simulink library "autolibshared"  (R2019b)
settings: Solver=ode45  StartTime=0.0  StopTime=10.0  RelTol=1e-3  EnableMultiTasking=on
undefined symbols (not defined in the file or in its folder): AccelCycle, aMode, DriveCycle, GearCycle, psi, x_o
libraries: autolibsharedcommon x20, $bdroot x7, autolibutils x2, autolibpowerinfoutils x1
(part 3 of 4)

== system autolibshared/Longitudinal Wheel/Longitudinal Parameters/Magic Formula Peak Value ==
  TirePrs : Inport
  Longitudinal Scaling : Inport  Port=2
  Bus Creator : BusCreator  Inputs=3
  Bus Creator1 : BusCreator  Inputs=5
  Bus Creator2 : BusCreator  Inputs=1
  Constant : Constant  Value=D
  Constant1 : Constant  Value=C
  Constant12 : Constant  Value=zeros(1,3)
  Constant14 : Constant  Value=zeros(3,3)
  Constant19 : Constant  Value=zeros(1,3)
  Constant2 : Constant  Value=zeros(34,1)
  Constant6 : Constant  Value=E
  Constant7 : Constant  Value=B
  Terminator : Terminator
  Magic Peak : Outport  VectorParamsAs1DForOutWhenUnconnected=off
  Magic Load Varying Fxo : Outport  Port=2  VectorParamsAs1DForOutWhenUnconnected=off
  Mapped Longitudinal Force : Outport  Port=3  VectorParamsAs1DForOutWhenUnconnected=off
  wires:
  Constant2/1 -> Bus Creator2/1
  Bus Creator2/1 -> Magic Load Varying Fxo/1
  Constant19/1 -> Bus Creator/1  "kappaFx"
  Constant12/1 -> Bus Creator/2  "FzFx"
  Constant14/1 -> Bus Creator/3  "FxMap"
  Longitudinal Scaling/1 -> Bus Creator1/5  "lam_mux"
  Bus Creator1/1 -> Magic Peak/1
  Bus Creator/1 -> Mapped Longitudinal Force/1  "mappedFx"
  Constant/1 -> Bus Creator1/1  "D"
  Constant1/1 -> Bus Creator1/2  "C"
  Constant6/1 -> Bus Creator1/4  "E"
  Constant7/1 -> Bus Creator1/3  "B"
  TirePrs/1 -> Terminator/1  "TirePrs"

== system autolibshared/Longitudinal Wheel/Longitudinal Parameters/Mapped Force ==
  TirePrs : Inport
  Longitudinal Scaling : Inport  Port=2
  Bus Creator : BusCreator  Inputs=3
  Bus Creator1 : BusCreator  Inputs=5
  Bus Creator2 : BusCreator  Inputs=1
  Constant{,1,6..7} (4 alike) : Constant  Value=0
  Constant12 : Constant  Value=FzFx
  Constant14 : Constant  Value=FxMap
  Constant19 : Constant  Value=kappaFx
  Constant2 : Constant  Value=zeros(34,1)
  Terminator : Terminator
  Magic Peak : Outport  VectorParamsAs1DForOutWhenUnconnected=off
  Magic Load Varying Fxo : Outport  Port=2  VectorParamsAs1DForOutWhenUnconnected=off
  Mapped Longitudinal Force : Outport  Port=3  VectorParamsAs1DForOutWhenUnconnected=off
  wires:
  Bus Creator2/1 -> Magic Load Varying Fxo/1
  Constant2/1 -> Bus Creator2/1
  Longitudinal Scaling/1 -> Bus Creator1/5  "lam_mux"
  Constant/1 -> Bus Creator1/1  "D"
  Constant6/1 -> Bus Creator1/4  "E"
  Bus Creator1/1 -> Magic Peak/1
  Constant7/1 -> Bus Creator1/3  "B"
  Constant1/1 -> Bus Creator1/2  "C"
  Constant19/1 -> Bus Creator/1  "kappaFx"
  Constant12/1 -> Bus Creator/2  "FzFx"
  Constant14/1 -> Bus Creator/3  "FxMap"
  Bus Creator/1 -> Mapped Longitudinal Force/1  "mappedFx"
  TirePrs/1 -> Terminator/1  "TirePrs"

== system autolibshared/Longitudinal Wheel/Rolling Parameters/ISO ==
  note: 8
  note: 16
  Temp : Inport  Unit=K
  Bus Creator : BusCreator  Inputs=3
  Bus Creator1 : BusCreator  Inputs=16
  Constant1 : Constant  Value=TMIN
  Constant{2,5,7,9..11,17..18} (8 alike) : Constant  Value=0
  Constant12 : Constant  Value=zeros(1,3)
  Constant13 : Constant  Value=Fpl
  Constant14 : Constant  Value=zeros(3,3)
  Constant15 : Constant  Value=Kt
  Constant16 : Constant  Value=Tmeas
  Constant19 : Constant  Value=zeros(1,3)
  Constant3 : Constant  Value=TMAX
  Constant4 : Constant  Value=UNLOADED_RADIUS
  Constant8 : Constant  Value=Cr
  Signal Specification{,1..3} (4 alike) : SignalSpecification  Unit=degC
  Signal Specification4 : SignalSpecification  Unit=K
  Signal Specification5 : SignalSpecification  Unit=K
  Signal Specification6 : SignalSpecification  Unit=K
  Unit Conversion{,1..3} (4 alike) : UnitConversion
  Magic Rolling Resistance : Outport  VectorParamsAs1DForOutWhenUnconnected=off
  Mapped Rolling Resistance : Outport  Port=2  VectorParamsAs1DForOutWhenUnconnected=off
  wires:
  Unit Conversion/1 -> Signal Specification/1
  Temp/1 -> Unit Conversion/1  "Temp"
  Constant10/1 -> Bus Creator1/13  "lam_My"
  Bus Creator1/1 -> Magic Rolling Resistance/1
  Constant18/1 -> Bus Creator1/11  "QSY8"
  Constant15/1 -> Bus Creator1/6  "QSY3"
  Constant17/1 -> Bus Creator1/10  "QSY7"
  Constant8/1 -> Bus Creator1/5  "QSY2"
  Constant5/1 -> Bus Creator1/2  "FNOMIN"
  Constant13/1 -> Bus Creator1/4  "QSY1"
  Constant2/1 -> Bus Creator1/3  "NOMPRES"
  Constant4/1 -> Bus Creator1/14  "UNLOADED_RADIUS"
  Signal Specification/1 -> Bus Creator1/1  "TAmb"
  Constant7/1 -> Bus Creator1/8  "QSY5"
  Constant9/1 -> Bus Creator1/9  "QSY6"
  Constant11/1 -> Bus Creator1/12  "gamma"
  Bus Creator/1 -> Mapped Rolling Resistance/1  "mappedMy"
  Constant14/1 -> Bus Creator/3  "MyMap"
  Constant12/1 -> Bus Creator/2  "FzMy"
  Constant19/1 -> Bus Creator/1  "VxMy"
  Unit Conversion1/1 -> Signal Specification1/1
  Signal Specification1/1 -> Bus Creator1/15  "TMin"
  Constant1/1 -> Signal Specification5/1
  Unit Conversion2/1 -> Signal Specification2/1
  Signal Specification2/1 -> Bus Creator1/16  "Tmax"
  Constant3/1 -> Signal Specification6/1
  Unit Conversion3/1 -> Signal Specification3/1
  Constant16/1 -> Signal Specification4/1
  Signal Specification3/1 -> Bus Creator1/7  "Tmeas"
  Signal Specification4/1 -> Unit Conversion3/1
  Signal Specification5/1 -> Unit Conversion1/1
  Signal Specification6/1 -> Unit Conversion2/1

== system autolibshared/Longitudinal Wheel/Rolling Parameters/Magic ==
  note: 8
  note: 16
  TirePrs : Inport  Unit=Pa
  Bus Creator : BusCreator  Inputs=3
  Bus Creator1 : BusCreator  Inputs=16
  Constant1 : Constant  Value=PRESMIN
  Constant10 : Constant  Value=lam_My
  Constant11 : Constant  Value=gamma
  Constant12 : Constant  Value=zeros(1,3)
  Constant13 : Constant  Value=QSY1
  Constant14 : Constant  Value=zeros(3,3)
  Constant15 : Constant  Value=QSY3
  Constant16 : Constant  Value=QSY4
  Constant17 : Constant  Value=QSY7
  Constant18 : Constant  Value=QSY8
  Constant19 : Constant  Value=zeros(1,3)
  Constant2 : Constant  Value=NOMPRES
  Constant3 : Constant  Value=PRESMAX
  Constant4 : Constant  Value=UNLOADED_RADIUS
  Constant5 : Constant  Value=FNOMIN
  Constant7 : Constant  Value=QSY5
  Constant8 : Constant  Value=QSY2
  Constant9 : Constant  Value=QSY6
  Magic Rolling Resistance : Outport  VectorParamsAs1DForOutWhenUnconnected=off
  Mapped Rolling Resistance : Outport  Port=2  VectorParamsAs1DForOutWhenUnconnected=off
  wires:
  Constant19/1 -> Bus Creator/1  "VxMy"
  Constant12/1 -> Bus Creator/2  "FzMy"
  Constant14/1 -> Bus Creator/3  "MyMap"
  Bus Creator/1 -> Mapped Rolling Resistance/1  "mappedMy"
  Constant11/1 -> Bus Creator1/12  "gamma"
  Constant9/1 -> Bus Creator1/9  "QSY6"
  Constant7/1 -> Bus Creator1/8  "QSY5"
  TirePrs/1 -> Bus Creator1/1  "TirePrs"
  Constant4/1 -> Bus Creator1/14  "UNLOADED_RADIUS"
  Constant3/1 -> Bus Creator1/16  "PRESMAX"
  Constant1/1 -> Bus Creator1/15  "PRESMIN"
  Constant2/1 -> Bus Creator1/3  "NOMPRES"
  Constant13/1 -> Bus Creator1/4  "QSY1"
  Constant5/1 -> Bus Creator1/2  "FNOMIN"
  Constant8/1 -> Bus Creator1/5  "QSY2"
  Constant17/1 -> Bus Creator1/10  "QSY7"
  Constant15/1 -> Bus Creator1/6  "QSY3"
  Constant16/1 -> Bus Creator1/7  "QSY4"
  Constant18/1 -> Bus Creator1/11  "QSY8"
  Bus Creator1/1 -> Magic Rolling Resistance/1
  Constant10/1 -> Bus Creator1/13  "lam_My"

== system autolibshared/Longitudinal Wheel/Rolling Parameters/Mapped ==
  TirePrs : Inport  Unit=Pa
  Bus Creator : BusCreator  Inputs=3
  Bus Creator1 : BusCreator  Inputs=16
  Constant{1..10,13,15..18} (15 alike) : Constant  Value=0
  Constant12 : Constant  Value=FzMy
  Constant14 : Constant  Value=MyMap
  Constant19 : Constant  Value=VxMy
  Magic Rolling Resistance : Outport  VectorParamsAs1DForOutWhenUnconnected=off
  Mapped Rolling Resistance : Outport  Port=2  VectorParamsAs1DForOutWhenUnconnected=off
  wires:
  Constant19/1 -> Bus Creator/1  "VxMy"
  Constant12/1 -> Bus Creator/2  "FzMy"
  Constant14/1 -> Bus Creator/3  "MyMap"
  Bus Creator/1 -> Mapped Rolling Resistance/1  "mappedMy"
  Constant6/1 -> Bus Creator1/12  "gamma"
  Constant9/1 -> Bus Creator1/9  "QSY6"
  Constant7/1 -> Bus Creator1/8  "QSY5"
  TirePrs/1 -> Bus Creator1/1  "TirePrs"
  Constant4/1 -> Bus Creator1/14  "UNLOADED_RADIUS"
  Constant3/1 -> Bus Creator1/16  "PRESMAX"
  Constant1/1 -> Bus Creator1/15  "PRESMIN"
  Constant2/1 -> Bus Creator1/3  "NOMPRES"
  Constant13/1 -> Bus Creator1/4  "QSY1"
  Constant5/1 -> Bus Creator1/2  "FNOMIN"
  Constant8/1 -> Bus Creator1/5  "QSY2"
  Constant17/1 -> Bus Creator1/10  "QSY7"
  Constant15/1 -> Bus Creator1/6  "QSY3"
  Constant16/1 -> Bus Creator1/7  "QSY4"
  Constant18/1 -> Bus Creator1/11  "QSY8"
  Bus Creator1/1 -> Magic Rolling Resistance/1
  Constant10/1 -> Bus Creator1/13  "lam_My"

== system autolibshared/Longitudinal Wheel/Rolling Parameters/None ==
  Bus Creator : BusCreator  Inputs=3
  Bus Creator1 : BusCreator  Inputs=16
  Constant{1,4,6..9,11,13,15..16} (10 alike) : Constant  Value=0
  Constant{2..3,5,10,17..18} (6 alike) : Constant
  Constant12 : Constant  Value=zeros(1,3)
  Constant14 : Constant  Value=zeros(3,3)
  Constant19 : Constant  Value=zeros(1,3)
  Magic Rolling Resistance : Outport  VectorParamsAs1DForOutWhenUnconnected=off
  Mapped Rolling Resistance : Outport  Port=2  VectorParamsAs1DForOutWhenUnconnected=off
  wires:
  Constant19/1 -> Bus Creator/1  "VxMy"
  Constant12/1 -> Bus Creator/2  "FzMy"
  Constant14/1 -> Bus Creator/3  "MyMap"
  Bus Creator/1 -> Mapped Rolling Resistance/1  "mappedMy"
  Constant6/1 -> Bus Creator1/12  "gamma"
  Constant9/1 -> Bus Creator1/9  "QSY6"
  Constant7/1 -> Bus Creator1/8  "QSY5"
  Constant11/1 -> Bus Creator1/1  "TirePrs"
  Constant4/1 -> Bus Creator1/14  "UNLOADED_RADIUS"
  Constant3/1 -> Bus Creator1/16  "PRESMAX"
  Constant1/1 -> Bus Creator1/15  "PRESMIN"
  Constant2/1 -> Bus Creator1/3  "NOMPRES"
  Constant13/1 -> Bus Creator1/4  "QSY1"
  Constant5/1 -> Bus Creator1/2  "FNOMIN"
  Constant8/1 -> Bus Creator1/5  "QSY2"
  Constant17/1 -> Bus Creator1/10  "QSY7"
  Constant15/1 -> Bus Creator1/6  "QSY3"
  Constant16/1 -> Bus Creator1/7  "QSY4"
  Constant18/1 -> Bus Creator1/11  "QSY8"
  Bus Creator1/1 -> Magic Rolling Resistance/1
  Constant10/1 -> Bus Creator1/13  "lam_My"

== system autolibshared/Longitudinal Wheel/Rolling Parameters/Simple ==
  note: 16
  note: 8
  TirePrs : Inport  Unit=Pa
  Bus Creator : BusCreator  Inputs=3
  Bus Creator1 : BusCreator  Inputs=16
  Constant1 : Constant  Value=PRESMIN
  Constant{2,5,7,9..11,16} (7 alike) : Constant  Value=0
  Constant12 : Constant  Value=zeros(1,3)
  Constant13 : Constant  Value=aMy
  Constant14 : Constant  Value=zeros(3,3)
  Constant15 : Constant  Value=cMy
  Constant17 : Constant  Value=betaMy
  Constant18 : Constant  Value=alphaMy
  Constant19 : Constant  Value=zeros(1,3)
  Constant3 : Constant  Value=PRESMAX
  Constant4 : Constant  Value=UNLOADED_RADIUS
  Constant8 : Constant  Value=bMy
  Magic Rolling Resistance : Outport  VectorParamsAs1DForOutWhenUnconnected=off
  Mapped Rolling Resistance : Outport  Port=2  VectorParamsAs1DForOutWhenUnconnected=off
  wires:
  Constant19/1 -> Bus Creator/1  "VxMy"
  Constant12/1 -> Bus Creator/2  "FzMy"
  Constant14/1 -> Bus Creator/3  "MyMap"
  Bus Creator/1 -> Mapped Rolling Resistance/1  "mappedMy"
  Constant11/1 -> Bus Creator1/12  "gamma"
  Constant9/1 -> Bus Creator1/9  "QSY6"
  Constant7/1 -> Bus Creator1/8  "QSY5"
  TirePrs/1 -> Bus Creator1/1  "TirePrs"
  Constant4/1 -> Bus Creator1/14  "UNLOADED_RADIUS"
  Constant3/1 -> Bus Creator1/16  "PRESMAX"
  Constant1/1 -> Bus Creator1/15  "PRESMIN"
  Constant2/1 -> Bus Creator1/3  "NOMPRES"
  Constant13/1 -> Bus Creator1/4  "QSY1"
  Constant5/1 -> Bus Creator1/2  "FNOMIN"
  Constant8/1 -> Bus Creator1/5  "QSY2"
  Constant17/1 -> Bus Creator1/10  "QSY7"
  Constant15/1 -> Bus Creator1/6  "QSY3"
  Constant16/1 -> Bus Creator1/7  "QSY4"
  Constant18/1 -> Bus Creator1/11  "QSY8"
  Bus Creator1/1 -> Magic Rolling Resistance/1
  Constant10/1 -> Bus Creator1/13  "lam_My"

== system autolibshared/Longitudinal Wheel/Vertical DOF/Magic Vertical DOF ==
  Fz : Inport
  Ground : Inport  Port=2
  FzTire : Inport  Port=3
  TirePrs : Inport  Port=4
  Bus Creator1 : BusCreator  Inputs=24
  Constant1 : Constant  Value=PRESMIN
  Constant10 : Constant  Value=Q_FCY
  Constant11 : Constant  Value=Q_FCY2
  Constant13 : Constant  Value=Q_CAM
  Constant14 : Constant  Value=NOMPRES
  Constant15 : Constant  Value=PFZ1
  Constant16 : Constant  Value=Q_CAM3
  Constant17 : Constant  Value=Q_FYS3
  Constant18 : Constant  Value=Q_FYS1
  Constant19 : Constant  Value=PRESMAX
  Constant2 : Constant  Value=VERTICAL_STIFFNESS
  Constant20 : Constant  Value=Q_FYS2
  Constant21 : Constant  Value=Q_CAM1
  Constant22 : Constant  Value=Q_CAM2
  Constant23 : Constant  Value=BOTTOM_STIFF
  Constant24 : Constant  Value=BOTTOM_OFFST
  Constant3 : Constant  Value=VERTICAL_DAMPING
  Constant4 : Constant  Value=Q_RE0
  Constant5 : Constant  Value=Q_V1
  Constant6 : Constant  Value=Q_V2
  Constant7 : Constant  Value=Q_FZ1
  Constant8 : Constant  Value=Q_FZ2
  Constant9 : Constant  Value=Q_FCX
  Signal Copy : SignalConversion  OverrideOpt=off
  Signal Copy1 : SignalConversion  OverrideOpt=off
  Vertical Wheel and Unsprung Mass Response : autolibsharedcommon/Vertical Wheel and Unsprung Mass Response  m=m  bz=VERTICAL_DAMPING  zo=zo  zdoto=zdoto  g=g
      settings: SourceProductName=Powertrain Blockset  SourceProductBaseCode=PW
  rhoz : Outport  VectorParamsAs1DForOutWhenUnconnected=off
  Fn : Outport  Port=2  VectorParamsAs1DForOutWhenUnconnected=off
  MagicVert : Outport  Port=3  VectorParamsAs1DForOutWhenUnconnected=off
  z : Outport  Port=4  VectorParamsAs1DForOutWhenUnconnected=off
  zdot : Outport  Port=5  VectorParamsAs1DForOutWhenUnconnected=off
  zddot : Outport  Port=6  VectorParamsAs1DForOutWhenUnconnected=off
  Fzb : Outport  Port=7  VectorParamsAs1DForOutWhenUnconnected=off
  Fzk : Outport  Port=8  VectorParamsAs1DForOutWhenUnconnected=off
  wires:
  Constant14/1 -> Bus Creator1/2  "NOMPRES"
  Constant1/1 -> Bus Creator1/3  "PRESMIN"
  Constant19/1 -> Bus Creator1/4  "PRESMAX"
  TirePrs/1 -> Bus Creator1/1  "TirePrs"
  Constant23/1 -> Bus Creator1/24  "BOTTOM_STIFF"
  Constant24/1 -> Bus Creator1/23  "BOTTOM_OFFST"
  Constant17/1 -> Bus Creator1/22  "Q_FYS3"
  Constant20/1 -> Bus Creator1/21  "Q_FYS2"
  Constant18/1 -> Bus Creator1/20  "Q_FYS1"
  Constant16/1 -> Bus Creator1/19  "Q_CAM3"
  Constant22/1 -> Bus Creator1/18  "Q_CAM2"
  Constant21/1 -> Bus Creator1/17  "Q_CAM1"
  Constant15/1 -> Bus Creator1/15  "PFZ1"
  Constant13/1 -> Bus Creator1/14  "Q_CAM"
  Constant11/1 -> Bus Creator1/16  "Q_FCY2"
  Constant8/1 -> Bus Creator1/11  "Q_FZ2"
  Constant9/1 -> Bus Creator1/12  "Q_FCX"
  Constant10/1 -> Bus Creator1/13  "Q_FCY"
  Constant7/1 -> Bus Creator1/10  "Q_FZ1"
  Constant6/1 -> Bus Creator1/9  "Q_V2"
  Constant5/1 -> Bus Creator1/8  "Q_V1"
  Constant4/1 -> Bus Creator1/7  "Q_RE0"
  Constant3/1 -> Bus Creator1/6  "VERTICAL_DAMPING"
  Bus Creator1/1 -> MagicVert/1  "magicFz"
  Constant2/1 -> Bus Creator1/5  "VERTICAL_STIFFNESS"
  Ground/1 -> Vertical Wheel and Unsprung Mass Response/1
  FzTire/1 -> Signal Copy1/1, Signal Copy/1, Vertical Wheel and Unsprung Mass Response/3
  Vertical Wheel and Unsprung Mass Response/3 -> zdot/1
  Vertical Wheel and Unsprung Mass Response/2 -> z/1
  Vertical Wheel and Unsprung Mass Response/1 -> rhoz/1
  Fz/1 -> Vertical Wheel and Unsprung Mass Response/2
  Vertical Wheel and Unsprung Mass Response/4 -> zddot/1
  Vertical Wheel and Unsprung Mass Response/5 -> Fzb/1
  Signal Copy/1 -> Fzk/1
  Signal Copy1/1 -> Fn/1

== system autolibshared/Longitudinal Wheel/Vertical DOF/Mapped Vertical DOF ==
  Fz : Inport
  Ground : Inport  Port=2
  FzTire : Inport  Port=3
  TirePrs : Inport  Port=4
  Bus Creator1 : BusCreator  Inputs=24
  Constant{1..24} (24 alike) : Constant  Value=0
  Terminator : Terminator
  Vertical Wheel and Unsprung Mass Mapped Response : autolibsharedcommon/Vertical Wheel and Unsprung Mass Mapped Response  m=m  zFz=zFz  zdotFz=zdotFz  Fzz=Fzz  pFz=pFz  Fzzdot=Fzzdot  zo=zo  zdoto=zdoto  g=g
      settings: SourceProductName=Powertrain Blockset  SourceProductBaseCode=PW
  rhoz : Outport  VectorParamsAs1DForOutWhenUnconnected=off
  Fn : Outport  Port=2  VectorParamsAs1DForOutWhenUnconnected=off
  MagicVert : Outport  Port=3  VectorParamsAs1DForOutWhenUnconnected=off
  z : Outport  Port=4  VectorParamsAs1DForOutWhenUnconnected=off
  zdot : Outport  Port=5  VectorParamsAs1DForOutWhenUnconnected=off
  zddot : Outport  Port=6  VectorParamsAs1DForOutWhenUnconnected=off
  Fzb : Outport  Port=7  VectorParamsAs1DForOutWhenUnconnected=off
  Fzk : Outport  Port=8  VectorParamsAs1DForOutWhenUnconnected=off
  wires:
  TirePrs/1 -> Vertical Wheel and Unsprung Mass Mapped Response/3
  Constant12/1 -> Bus Creator1/1  "press"
  Constant1/1 -> Bus Creator1/3  "PRESMIN"
  Constant19/1 -> Bus Creator1/4  "PRESMAX"
  Constant14/1 -> Bus Creator1/2  "NOMPRES"
  Vertical Wheel and Unsprung Mass Mapped Response/4 -> Fn/1
  FzTire/1 -> Terminator/1
  Constant23/1 -> Bus Creator1/24  "BOTTOM_STIFF"
  Constant24/1 -> Bus Creator1/23  "BOTTOM_OFFST"
  Constant20/1 -> Bus Creator1/22  "Q_FYS3"
  Constant18/1 -> Bus Creator1/21  "Q_FYS2"
  Constant22/1 -> Bus Creator1/20  "Q_FYS1"
  Constant21/1 -> Bus Creator1/19  "Q_CAM3"
  Constant15/1 -> Bus Creator1/18  "Q_CAM2"
  Constant13/1 -> Bus Creator1/17  "Q_CAM1"
  Constant16/1 -> Bus Creator1/15  "PFZ1"
  Constant11/1 -> Bus Creator1/14  "Q_CAM"
  Constant17/1 -> Bus Creator1/16  "Q_FCY2"
  Constant8/1 -> Bus Creator1/11  "Q_FZ2"
  Constant9/1 -> Bus Creator1/12  "Q_FCX"
  Constant10/1 -> Bus Creator1/13  "Q_FCY"
  Constant7/1 -> Bus Creator1/10  "Q_FZ1"
  Constant6/1 -> Bus Creator1/9  "Q_V2"
  Constant5/1 -> Bus Creator1/8  "Q_V1"
  Constant4/1 -> Bus Creator1/7  "Q_RE0"
  Constant3/1 -> Bus Creator1/6  "VERTICAL_DAMPING"
  Bus Creator1/1 -> MagicVert/1  "magicFz"
  Constant2/1 -> Bus Creator1/5  "VERTICAL_STIFFNESS"
  Ground/1 -> Vertical Wheel and Unsprung Mass Mapped Response/1
  Vertical Wheel and Unsprung Mass Mapped Response/3 -> zdot/1
  Vertical Wheel and Unsprung Mass Mapped Response/2 -> z/1
  Vertical Wheel and Unsprung Mass Mapped Response/1 -> rhoz/1
  Fz/1 -> Vertical Wheel and Unsprung Mass Mapped Response/2
  Vertical Wheel and Unsprung Mass Mapped Response/5 -> zddot/1
  Vertical Wheel and Unsprung Mass Mapped Response/7 -> Fzk/1
  Vertical Wheel and Unsprung Mass Mapped Response/6 -> Fzb/1

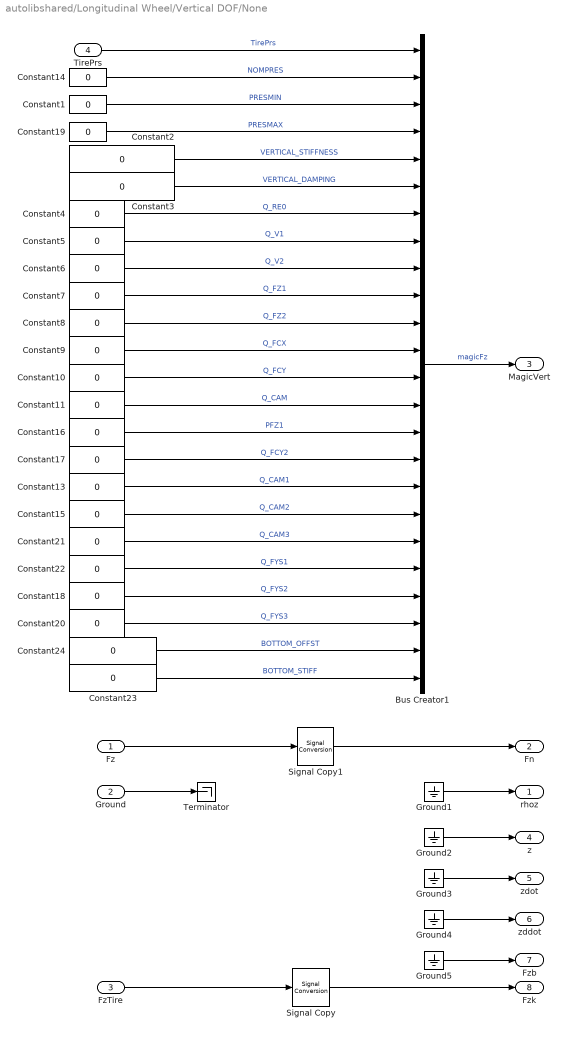
== system autolibshared/Longitudinal Wheel/Vertical DOF/None ==
  Fz : Inport
  Ground : Inport  Port=2
  FzTire : Inport  Port=3
  TirePrs : Inport  Port=4
  Bus Creator1 : BusCreator  Inputs=24
  Constant{1..11,13..24} (23 alike) : Constant  Value=0
  Ground{1..5} (5 alike) : Ground
  Signal Copy : SignalConversion  OverrideOpt=off
  Signal Copy1 : SignalConversion  OverrideOpt=off
  Terminator : Terminator
  rhoz : Outport  VectorParamsAs1DForOutWhenUnconnected=off
  Fn : Outport  Port=2  VectorParamsAs1DForOutWhenUnconnected=off
  MagicVert : Outport  Port=3  VectorParamsAs1DForOutWhenUnconnected=off
  z : Outport  Port=4  PortDimensions=1  VectorParamsAs1DForOutWhenUnconnected=off
  zdot : Outport  Port=5  PortDimensions=1  VectorParamsAs1DForOutWhenUnconnected=off
  zddot : Outport  Port=6  PortDimensions=1  VectorParamsAs1DForOutWhenUnconnected=off
  Fzb : Outport  Port=7  PortDimensions=1  VectorParamsAs1DForOutWhenUnconnected=off
  Fzk : Outport  Port=8  VectorParamsAs1DForOutWhenUnconnected=off
  wires:
  Bus Creator1/1 -> MagicVert/1  "magicFz"
  Constant1/1 -> Bus Creator1/3  "PRESMIN"
  TirePrs/1 -> Bus Creator1/1  "TirePrs"
  Constant14/1 -> Bus Creator1/2  "NOMPRES"
  Constant9/1 -> Bus Creator1/12  "Q_FCX"
  Constant3/1 -> Bus Creator1/6  "VERTICAL_DAMPING"
  Constant4/1 -> Bus Creator1/7  "Q_RE0"
  Constant19/1 -> Bus Creator1/4  "PRESMAX"
  Constant16/1 -> Bus Creator1/15  "PFZ1"
  Constant5/1 -> Bus Creator1/8  "Q_V1"
  Constant6/1 -> Bus Creator1/9  "Q_V2"
  Constant24/1 -> Bus Creator1/23  "BOTTOM_OFFST"
  Constant2/1 -> Bus Creator1/5  "VERTICAL_STIFFNESS"
  Constant11/1 -> Bus Creator1/14  "Q_CAM"
  Constant17/1 -> Bus Creator1/16  "Q_FCY2"
  Constant8/1 -> Bus Creator1/11  "Q_FZ2"
  Constant7/1 -> Bus Creator1/10  "Q_FZ1"
  Constant10/1 -> Bus Creator1/13  "Q_FCY"
  Constant13/1 -> Bus Creator1/17  "Q_CAM1"
  Constant21/1 -> Bus Creator1/19  "Q_CAM3"
  Constant20/1 -> Bus Creator1/22  "Q_FYS3"
  Constant15/1 -> Bus Creator1/18  "Q_CAM2"
  Constant23/1 -> Bus Creator1/24  "BOTTOM_STIFF"
  Constant18/1 -> Bus Creator1/21  "Q_FYS2"
  Constant22/1 -> Bus Creator1/20  "Q_FYS1"
  Fz/1 -> Signal Copy1/1
  Ground/1 -> Terminator/1
  Ground3/1 -> zdot/1
  Ground2/1 -> z/1
  Ground1/1 -> rhoz/1
  Ground4/1 -> zddot/1
  FzTire/1 -> Signal Copy/1
  Ground5/1 -> Fzb/1
  Signal Copy/1 -> Fzk/1
  Signal Copy1/1 -> Fn/1

== system autolibshared/Longitudinal Wheel/Wheel Module/Brakes ==
  note: 1) Add Subsystem or Model blocks as valid variant choices.
      | 2) You cannot connect blocks at this level. At simulation, connectivity is automatically
      | determined, based on the active variant and port name matching.
  BrkPrs : Inport
  Omega : Inport  Port=2
  Disk Brake : Subsystem  VariantControl=Disk
  Drum Brake : Subsystem  VariantControl=Drum
  Mapped Brake : Subsystem  VariantControl=Mapped
  No Brake : Subsystem  VariantControl=None
  MyBrk : Outport  VectorParamsAs1DForOutWhenUnconnected=off

== system autolibshared/Longitudinal Wheel/Wheel Module/Clutch/Locked ==
  Tout : Inport
  f : ActionPort
      settings: CopyFcn=Stateflow.SLINSF.SimulinkMan.removeBlockPreDeleteFcn  PreDeleteFcn=Stateflow.SLINSF.SimulinkMan.unsafePredeleteFcn
  Unary Minus : UnaryMinus
  locked : Constant  Value=0
  locked1 : Constant  Value=0
  locked2 : Constant  Value=0
  ReactionTorque : Outport  InitialOutput=0  VectorParamsAs1DForOutWhenUnconnected=off
  Omega : Outport  Port=2  InitialOutput=0  VectorParamsAs1DForOutWhenUnconnected=off
  Omegadot : Outport  Port=3  InitialOutput=0  VectorParamsAs1DForOutWhenUnconnected=off
  Myb : Outport  Port=4  InitialOutput=0  VectorParamsAs1DForOutWhenUnconnected=off
  wires:
  Unary Minus/1 -> ReactionTorque/1
  locked1/1 -> Omegadot/1
  locked/1 -> Omega/1
  Tout/1 -> Unary Minus/1
  locked2/1 -> Myb/1

== system autolibshared/Longitudinal Wheel/Wheel Module/Clutch/Slipping ==
  Tfmaxk : Inport
  Tout : Inport  Port=2
  f : ActionPort
      settings: CopyFcn=Stateflow.SLINSF.SimulinkMan.removeBlockPreDeleteFcn  PreDeleteFcn=Stateflow.SLINSF.SimulinkMan.unsafePredeleteFcn
  -4 : Gain  Gain=-4  SaturateOnIntegerOverflow=on  OutDataTypeStr=Inherit: Same as input  ParamDataTypeStr=Inherit: Same as input
  Max Dynamic Friction Torque1 : Product  SaturateOnIntegerOverflow=on  RndMeth=Zero  InputSameDT=on  OutDataTypeStr=Inherit: Same as first input
  Output Inertia : Gain  Gain=1./0.82  SaturateOnIntegerOverflow=on  OutDataTypeStr=Inherit: Same as input  ParamDataTypeStr=Inherit: Same as input
  Output Damping : Gain  Gain=1e-3  SaturateOnIntegerOverflow=on  OutDataTypeStr=Inherit: Same as input  ParamDataTypeStr=Inherit: Same as input
  Output Sum : Sum  Inputs=|+--  SaturateOnIntegerOverflow=on  InputSameDT=on  OutDataTypeStr=Inherit: Same as first input
  Trigonometric Function : Trigonometry  Operator=tanh
  omega wheel : Integrator  ContinuousStateAttributes='omegaWheel'
  Omega : Outport  InitialOutput=0  VectorParamsAs1DForOutWhenUnconnected=off
  Omegadot : Outport  Port=2  InitialOutput=0  VectorParamsAs1DForOutWhenUnconnected=off
  ReactionTorque : Outport  Port=3  InitialOutput=0  VectorParamsAs1DForOutWhenUnconnected=off
  Myb : Outport  Port=4  InitialOutput=0  VectorParamsAs1DForOutWhenUnconnected=off
  wires:
  Output Damping/1 -> Myb/1, Output Sum/3
  omega wheel/1 -> Omega/1, -4/1, Output Damping/1
  Output Sum/1 -> ReactionTorque/1, Output Inertia/1
  Tout/1 -> Output Sum/2
  Max Dynamic Friction Torque1/1 -> Output Sum/1
  Trigonometric Function/1 -> Max Dynamic Friction Torque1/2
  -4/1 -> Trigonometric Function/1
  Output Inertia/1 -> Omegadot/1, omega wheel/1
  Tfmaxk/1 -> Max Dynamic Friction Torque1/1

== system autolibshared/Longitudinal Wheel/Wheel Module/Clutch/detectLockup ==
  Tout : Inport
  Tfmaxs : Inport  Port=2
  f : TriggerPort  TriggerType=function-call  VariantControl=Variant
      settings: CopyFcn=Stateflow.SLINSF.SimulinkMan.removeBlockPreDeleteFcn  PreDeleteFcn=Stateflow.SLINSF.SimulinkMan.unsafePredeleteFcn
  Constant : Constant  Value=0
  Friction Mode Logic : Subsystem
      mask Display: plot([-3 1 1 3 -1 -1],[-1 -1 1 1 1 -1],-4,-5,4,5)
  yn : Outport  VectorParamsAs1DForOutWhenUnconnected=off
  wires:
  Tfmaxs/1 -> Friction Mode Logic/2(Tfmaxs)
  Tout/1 -> Friction Mode Logic/1(Tout)
  Friction Mode Logic/1(locked) -> yn/1  "LockedFlag"
  Constant/1 -> Friction Mode Logic/3(locked_wout)

== system autolibshared/Longitudinal Wheel/Wheel Module/Clutch/detectSlip ==
  Tout : Inport
  Tfmaxs : Inport  Port=2
  f : TriggerPort  TriggerType=function-call  VariantControl=Variant
      settings: CopyFcn=Stateflow.SLINSF.SimulinkMan.removeBlockPreDeleteFcn  PreDeleteFcn=Stateflow.SLINSF.SimulinkMan.unsafePredeleteFcn
  Break Apart Detection : Subsystem
  yn : Outport  VectorParamsAs1DForOutWhenUnconnected=off
  wires:
  Tfmaxs/1 -> Break Apart Detection/1(Tfmaxs)
  Tout/1 -> Break Apart Detection/2(Tf)
  Break Apart Detection/1(unlock) -> yn/1

== system autolibshared/Longitudinal Wheel/Wheel Module/Friction Model ==
  Brake torque : Inport
  Ratio of static to kinetic : Gain  Gain=0.3/0.2  SaturateOnIntegerOverflow=on  OutDataTypeStr=Inherit: Same as input  ParamDataTypeStr=Inherit: Same as input
  Tfmaxs : Outport  InitialOutput=0  VectorParamsAs1DForOutWhenUnconnected=off
  Tfmaxk : Outport  Port=2  InitialOutput=0  VectorParamsAs1DForOutWhenUnconnected=off
  wires:
  Brake torque/1 -> Tfmaxk/1, Ratio of static to kinetic/1
  Ratio of static to kinetic/1 -> Tfmaxs/1

== system autolibshared/Vehicle Body 3DOF Single Track/Cy/Cy const ==
  Cyf : Constant  Value=Cy_f
  Cyr : Constant  Value=Cy_r
  Cy_f : Outport  VectorParamsAs1DForOutWhenUnconnected=off
  Cy_r : Outport  Port=2  VectorParamsAs1DForOutWhenUnconnected=off
  wires:
  Cyf/1 -> Cy_f/1
  Cyr/1 -> Cy_r/1

== system autolibshared/Vehicle Body 3DOF Single Track/Cy/Cy const dual ==
  Cyf : Constant  Value=Cy_f
  Cyr : Constant  Value=Cy_r
  Vector Concatenate1 : Concatenate
  Vector Concatenate2 : Concatenate  ConcatenateDimension=2
  Cy_f : Outport  VectorParamsAs1DForOutWhenUnconnected=off
  Cy_r : Outport  Port=2  VectorParamsAs1DForOutWhenUnconnected=off
  wires:
  Vector Concatenate1/1 -> Cy_r/1
  Vector Concatenate2/1 -> Cy_f/1
  Cyr/1 -> Vector Concatenate1/1, Vector Concatenate1/2
  Cyf/1 -> Vector Concatenate2/1, Vector Concatenate2/2

== system autolibshared/Vehicle Body 3DOF Single Track/Cy/Cy table ==
  alpha_f : Inport
  alpha_r : Inport  Port=2
  Cy_f(alpha_f) : Lookup_n-D  NumberOfTableDimensions=1  BreakpointsForDimension1=alpha_f_brk  Table=Cy_f_data  ExtrapMethod=Clip  InternalRulePriority=Speed  RndMeth=Simplest  InputSameDT=on
  Cy_r(alpha_r) : Lookup_n-D  NumberOfTableDimensions=1  BreakpointsForDimension1=alpha_r_brk  Table=Cy_r_data  ExtrapMethod=Clip  InternalRulePriority=Speed  RndMeth=Simplest  InputSameDT=on
  Cy_f : Outport  VectorParamsAs1DForOutWhenUnconnected=off
  Cy_r : Outport  Port=2  VectorParamsAs1DForOutWhenUnconnected=off
  wires:
  Cy_f(alpha_f)/1 -> Cy_f/1
  Cy_r(alpha_r)/1 -> Cy_r/1
  alpha_f/1 -> Cy_f(alpha_f)/1
  alpha_r/1 -> Cy_r(alpha_r)/1

== system autolibshared/Vehicle Body 3DOF Single Track/Cy/Cy table dual ==
  alpha_f : Inport
  alpha_r : Inport  Port=2
  For Each Subsystem : Subsystem  TreatAsAtomicUnit=on
  Cy_f : Outport  VectorParamsAs1DForOutWhenUnconnected=off
  Cy_r : Outport  Port=2  VectorParamsAs1DForOutWhenUnconnected=off
  wires:
  For Each Subsystem/1(Cy_f) -> Cy_f/1
  For Each Subsystem/2(Cy_r) -> Cy_r/1
  alpha_f/1 -> For Each Subsystem/1(alpha_f)
  alpha_r/1 -> For Each Subsystem/2(alpha_r)

== system autolibshared/Vehicle Body 3DOF Single Track/Drag/inertial2body ==
  psi : Inport
  WindXYZ : Inport  Port=2
  Add : Sum
  Add1 : Sum  Inputs=-+
  Demux1 : Demux  Outputs=3
  Product{,1..3} (4 alike) : Product
  Trigonometric Function : Trigonometry  Operator=sincos
  Vector Concatenate2 : Concatenate  NumInputs=3
  Windxyz : Outport  VectorParamsAs1DForOutWhenUnconnected=off
  wires:
  Demux1/2 -> Product2/2, Product1/2
  Demux1/1 -> Product3/2, Product/2
  Trigonometric Function/2 -> Product3/1, Product2/1
  Trigonometric Function/1 -> Product1/1, Product/1
  Product2/1 -> Add1/2
  Product/1 -> Add1/1
  Vector Concatenate2/1 -> Windxyz/1
  Add1/1 -> Vector Concatenate2/2
  Add/1 -> Vector Concatenate2/1
  Product3/1 -> Add/1
  Demux1/3 -> Vector Concatenate2/3
  Product1/1 -> Add/2
  WindXYZ/1 -> Demux1/1
  psi/1 -> Trigonometric Function/1

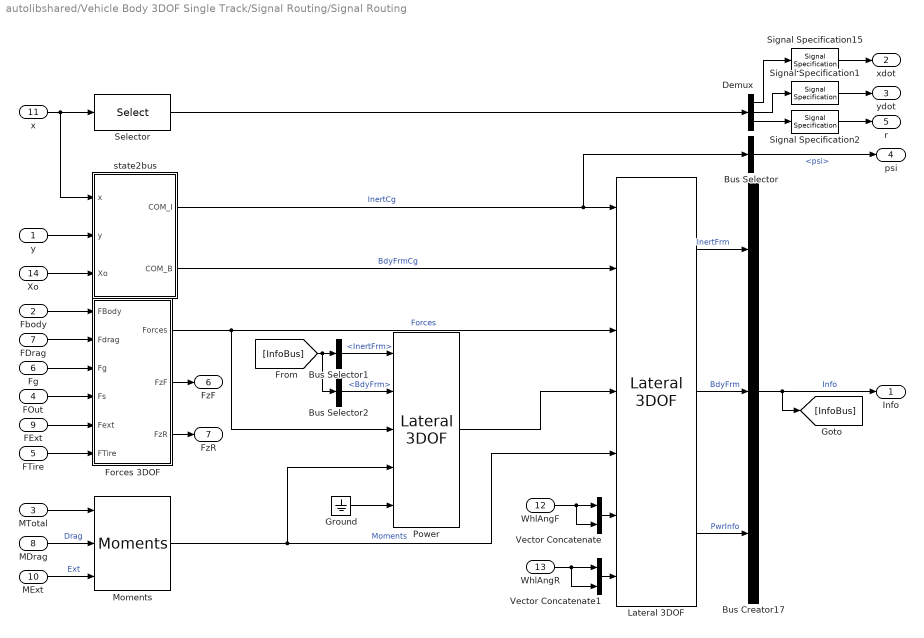
== system autolibshared/Vehicle Body 3DOF Single Track/Signal Routing/Signal Routing ==
  y : Inport  PortDimensions=3
  Fbody : Inport  Port=2
  MTotal : Inport  Port=3
  FOut : Inport  Port=4  PortDimensions=6
  FTire : Inport  Port=5
  Fg : Inport  Port=6
  FDrag : Inport  Port=7
  MDrag : Inport  Port=8
  FExt : Inport  Port=9
  MExt : Inport  Port=10
  x : Inport  Port=11
  WhlAngF : Inport  Port=12
  WhlAngR : Inport  Port=13
  Xo : Inport  Port=14
  Bus Creator17 : BusCreator  Inputs=3
  Bus Selector : BusSelector  OutputSignals=Ang.psi
  Bus Selector1 : BusSelector  OutputSignals=InertFrm
  Bus Selector2 : BusSelector  OutputSignals=BdyFrm
  Demux : Demux  Outputs=3
  Forces 3DOF : Subsystem  VariantControl=2
  Ground : Ground
  Lateral 3DOF : autolibsharedcommon/Bus Creation/Frame Routing/Lateral 3DOF  VariantControl=3  aMode=aMode
      settings: SourceProductName=Powertrain Blockset  SourceProductBaseCode=PW
  Moments : autolibsharedcommon/Bus Creation/Moments  SystemSampleTime=-1  Latency=0  AutoFrameSizeCalculation=off
      settings: SourceProductName=Powertrain Blockset  SourceProductBaseCode=PW
  Power : autolibsharedcommon/Bus Creation/Power/Lateral 3DOF  SystemSampleTime=-1  VariantControl=3  Latency=0  AutoFrameSizeCalculation=off
      settings: SourceProductName=Powertrain Blockset  SourceProductBaseCode=PW
  Selector : Selector  IndexOptions=Index vector (dialog)  Indices=[1,2,4]  OutputSizes=1
  Signal Specification1 : SignalSpecification  Unit=m/s
  Signal Specification15 : SignalSpecification  Unit=m/s
  Signal Specification2 : SignalSpecification  Unit=rad/s
  Vector Concatenate : Concatenate
  Vector Concatenate1 : Concatenate
  state2bus : Subsystem
  Info : Outport  VectorParamsAs1DForOutWhenUnconnected=off
  xdot : Outport  Port=2  VectorParamsAs1DForOutWhenUnconnected=off
  ydot : Outport  Port=3  VectorParamsAs1DForOutWhenUnconnected=off
  psi : Outport  Port=4  VectorParamsAs1DForOutWhenUnconnected=off
  r : Outport  Port=5  VectorParamsAs1DForOutWhenUnconnected=off
  FzF : Outport  Port=6  VectorParamsAs1DForOutWhenUnconnected=off
  FzR : Outport  Port=7  VectorParamsAs1DForOutWhenUnconnected=off
  wires:
  MTotal/1 -> Moments/1
  MDrag/1 -> Moments/2  "Drag"
  Fbody/1 -> Forces 3DOF/1(FBody)
  Power/1 -> Lateral 3DOF/4
  MExt/1 -> Moments/3  "Ext"
  Moments/1 -> Power/4, Lateral 3DOF/5  "Moments"
  FExt/1 -> Forces 3DOF/5(Fext)
  Forces 3DOF/3(FzR) -> FzR/1
  Forces 3DOF/2(FzF) -> FzF/1
  FDrag/1 -> Forces 3DOF/2(Fdrag)
  FOut/1 -> Forces 3DOF/4(Fs)
  Forces 3DOF/1(Forces) -> Power/3, Lateral 3DOF/3  "Forces"
  FTire/1 -> Forces 3DOF/6(FTire)
  Fg/1 -> Forces 3DOF/3(Fg)
  Lateral 3DOF/2 -> Bus Creator17/2  "BdyFrm"
  Signal Specification2/1 -> r/1
  Signal Specification1/1 -> ydot/1
  Signal Specification15/1 -> xdot/1
  x/1 -> state2bus/1(x), Selector/1
  Demux/3 -> Signal Specification2/1
  Demux/2 -> Signal Specification1/1
  Demux/1 -> Signal Specification15/1
  Selector/1 -> Demux/1
  y/1 -> state2bus/2(y)
  Bus Creator17/1 -> [InfoBus], Info/1  "Info"
  Lateral 3DOF/1 -> Bus Creator17/1  "InertFrm"
  state2bus/1(COM_I) -> Bus Selector/1, Lateral 3DOF/1  "InertCg"
  state2bus/2(COM_B) -> Lateral 3DOF/2  "BdyFrmCg"
  WhlAngR/1 -> Vector Concatenate1/2, Vector Concatenate1/1
  WhlAngF/1 -> Vector Concatenate/2, Vector Concatenate/1
  Vector Concatenate/1 -> Lateral 3DOF/6
  Vector Concatenate1/1 -> Lateral 3DOF/7
  Xo/1 -> state2bus/3(Xo)
  Lateral 3DOF/3 -> Bus Creator17/3  "PwrInfo"
  [InfoBus] -> Bus Selector1/1, Bus Selector2/1
  Bus Selector1/1 -> Power/1  "<InertFrm>"
  Bus Selector2/1 -> Power/2  "<BdyFrm>"
  Ground/1 -> Power/5
  Bus Selector/1 -> psi/1  "<psi>"

== system autolibshared/Vehicle Body 3DOF Single Track/Signal Routing/Signal Routing Dual ==
  y : Inport
  Fbody : Inport  Port=2
  MTotal : Inport  Port=3
  FOut : Inport  Port=4
  FTire : Inport  Port=5
  Fg : Inport  Port=6
  FDrag : Inport  Port=7
  MDrag : Inport  Port=8
  FExt : Inport  Port=9
  MExt : Inport  Port=10
  x : Inport  Port=11
  WhlAngF : Inport  Port=12
  WhlAngR : Inport  Port=13
  Xo : Inport  Port=14
  Bus Creator17 : BusCreator  Inputs=3
  Bus Selector : BusSelector  OutputSignals=Ang.psi
  Bus Selector1 : BusSelector  OutputSignals=InertFrm
  Bus Selector2 : BusSelector  OutputSignals=BdyFrm
  Demux : Demux  Outputs=3
  Forces 3DOF : Subsystem  VariantControl=2
  Ground : Ground
  Lateral 3DOF : Subsystem  VariantControl=2
  Moments : autolibsharedcommon/Bus Creation/Moments  SystemSampleTime=-1  Latency=0  AutoFrameSizeCalculation=off
      settings: SourceProductName=Powertrain Blockset  SourceProductBaseCode=PW
  Power : autolibsharedcommon/Bus Creation/Power/Lateral 3DOF Dual  SystemSampleTime=-1  VariantControl=4  Latency=0  AutoFrameSizeCalculation=off
      settings: SourceProductName=Powertrain Blockset  SourceProductBaseCode=PW
  Selector : Selector  IndexOptions=Index vector (dialog)  Indices=[1,2,4]  OutputSizes=1
  Signal Specification1 : SignalSpecification  Unit=m/s
  Signal Specification15 : SignalSpecification  Unit=m/s
  Signal Specification2 : SignalSpecification  Unit=rad/s
  state2bus : Subsystem
  Info : Outport  VectorParamsAs1DForOutWhenUnconnected=off
  xdot : Outport  Port=2  VectorParamsAs1DForOutWhenUnconnected=off
  ydot : Outport  Port=3  VectorParamsAs1DForOutWhenUnconnected=off
  psi : Outport  Port=4  VectorParamsAs1DForOutWhenUnconnected=off
  r : Outport  Port=5  VectorParamsAs1DForOutWhenUnconnected=off
  FzF : Outport  Port=6  VectorParamsAs1DForOutWhenUnconnected=off
  FzR : Outport  Port=7  VectorParamsAs1DForOutWhenUnconnected=off
  wires:
  Lateral 3DOF/1(InertFrm) -> Bus Creator17/1  "InertFrm"
  Bus Creator17/1 -> [InfoBus], Info/1  "Info"
  y/1 -> state2bus/2(y)
  Selector/1 -> Demux/1
  Demux/1 -> Signal Specification15/1
  Demux/2 -> Signal Specification1/1
  state2bus/1(COM_I) -> Lateral 3DOF/1(InertCg), Bus Selector/1  "InertCg"
  state2bus/2(COM_B) -> Lateral 3DOF/2(BdyFrmCg)  "BdyFrmCg"
  x/1 -> Selector/1, state2bus/1(x)
  Signal Specification15/1 -> xdot/1
  Signal Specification1/1 -> ydot/1
  Signal Specification2/1 -> r/1
  Lateral 3DOF/2(BdyFrm) -> Bus Creator17/2  "BdyFrm"
  Fg/1 -> Forces 3DOF/3(Fg)
  FTire/1 -> Forces 3DOF/6(FTire)
  Forces 3DOF/1(Forces) -> Power/3, Lateral 3DOF/3(Forces)  "Forces"
  FOut/1 -> Forces 3DOF/4(Fs)
  FDrag/1 -> Forces 3DOF/2(Fdrag)
  Forces 3DOF/2(FzF) -> FzF/1
  Forces 3DOF/3(FzR) -> FzR/1
  FExt/1 -> Forces 3DOF/5(Fext)
  Moments/1 -> Power/4, Lateral 3DOF/5(Moments)  "Moments"
  MExt/1 -> Moments/3  "Ext"
  Power/1 -> Lateral 3DOF/4(Power)
  Fbody/1 -> Forces 3DOF/1(FBody)
  MDrag/1 -> Moments/2  "Drag"
  MTotal/1 -> Moments/1
  WhlAngF/1 -> Lateral 3DOF/6(WhlAngF)
  WhlAngR/1 -> Lateral 3DOF/7(WhlAngR)
  Xo/1 -> state2bus/3(Xo)
  Bus Selector2/1 -> Power/2  "<BdyFrm>"
  [InfoBus] -> Bus Selector1/1, Bus Selector2/1
  Bus Selector1/1 -> Power/1  "<InertFrm>"
  Lateral 3DOF/3(PwrInfo) -> Bus Creator17/3  "PwrInfo"
  Ground/1 -> Power/5
  Demux/3 -> Signal Specification2/1
  Bus Selector/1 -> psi/1  "<psi>"

== system autolibshared/Vehicle Body 3DOF Single Track/friction/mu ext ==
  mu_in : Inport  Unit=1
  Signal Specification1 : SignalSpecification  Unit=1
  Unit Conversion2 : UnitConversion
  mu_out : Outport  Unit=1  VectorParamsAs1DForOutWhenUnconnected=off
  wires:
  Unit Conversion2/1 -> Signal Specification1/1
  mu_in/1 -> Unit Conversion2/1
  Signal Specification1/1 -> mu_out/1

== system autolibshared/Vehicle Body 3DOF Single Track/friction/mu ext dual ==
  mu_in : Inport  PortDimensions=[2,2]
  Signal Specification1 : SignalSpecification  Unit=1
  Unit Conversion2 : UnitConversion
  mu_out : Outport  PortDimensions=[2,2]  VectorParamsAs1DForOutWhenUnconnected=off
  wires:
  Unit Conversion2/1 -> Signal Specification1/1
  mu_in/1 -> Unit Conversion2/1
  Signal Specification1/1 -> mu_out/1

== system autolibshared/Vehicle Body 3DOF Single Track/friction/mu int ==
  Constant : Constant  Value=mu
  Vector Concatenate1 : Concatenate
  mu_out : Outport  VectorParamsAs1DForOutWhenUnconnected=off
  wires:
  Vector Concatenate1/1 -> mu_out/1
  Constant/1 -> Vector Concatenate1/2, Vector Concatenate1/1

== system autolibshared/Vehicle Body 3DOF Single Track/friction/mu int dual ==
  Constant : Constant  Value=mu
  Vector Concatenate2 : Concatenate  Mode=Multidimensional array  ConcatenateDimension=2
  Vector Concatenate3 : Concatenate  Mode=Multidimensional array  ConcatenateDimension=2
  Vector Concatenate4 : Concatenate  Mode=Multidimensional array
  mu_out : Outport  VectorParamsAs1DForOutWhenUnconnected=off
  wires:
  Constant/1 -> Vector Concatenate2/1, Vector Concatenate2/2, Vector Concatenate3/1, Vector Concatenate3/2
  Vector Concatenate4/1 -> mu_out/1
  Vector Concatenate3/1 -> Vector Concatenate4/2
  Vector Concatenate2/1 -> Vector Concatenate4/1

== system autolibshared/Vehicle Body 3DOF Single Track/front forces/ext ==
  F_in : Inport  PortDimensions=2
  Signal Specification1 : SignalSpecification  Unit=N
  Unit Conversion3 : UnitConversion
  F_out : Outport  Unit=N  VectorParamsAs1DForOutWhenUnconnected=off
  wires:
  Unit Conversion3/1 -> Signal Specification1/1
  F_in/1 -> Unit Conversion3/1
  Signal Specification1/1 -> F_out/1

== system autolibshared/Vehicle Body 3DOF Single Track/front forces/ext dual ==
  F_in : Inport  PortDimensions=[2,2]
  Signal Specification1 : SignalSpecification  Unit=N
  Unit Conversion3 : UnitConversion
  F_out : Outport  Unit=N  PortDimensions=[2,2]  VectorParamsAs1DForOutWhenUnconnected=off
  wires:
  Unit Conversion3/1 -> Signal Specification1/1
  F_in/1 -> Unit Conversion3/1
  Signal Specification1/1 -> F_out/1

== system autolibshared/Vehicle Body 3DOF Single Track/front forces/ext long ==
  F_in : Inport
  Ground1 : Ground
  Signal Specification : SignalSpecification  Unit=N
  Signal Specification1 : SignalSpecification  Unit=N
  Unit Conversion1 : UnitConversion
  Vector Concatenate1 : Concatenate
  F_out : Outport  Unit=N  VectorParamsAs1DForOutWhenUnconnected=off
  wires:
  Signal Specification1/1 -> Vector Concatenate1/1
  Unit Conversion1/1 -> Signal Specification1/1
  Ground1/1 -> Signal Specification/1
  Vector Concatenate1/1 -> F_out/1
  F_in/1 -> Unit Conversion1/1
  Signal Specification/1 -> Vector Concatenate1/2

== system autolibshared/Vehicle Body 3DOF Single Track/front forces/ext long dual ==
  F_in : Inport
  Demux : Demux  Outputs=2
  Ground : Ground
  Signal Specification5 : SignalSpecification  Unit=N
  Unit Conversion2 : UnitConversion  OutputType=Inherit: Inherit via back propagation
  Vector Concatenate1 : Concatenate  Mode=Multidimensional array  ConcatenateDimension=2
  Vector Concatenate2 : Concatenate  Mode=Multidimensional array  ConcatenateDimension=2
  Vector Concatenate3 : Concatenate  Mode=Multidimensional array
  F_out : Outport  Unit=N  VectorParamsAs1DForOutWhenUnconnected=off
  wires:
  F_in/1 -> Unit Conversion2/1
  Signal Specification5/1 -> Demux/1
  Unit Conversion2/1 -> Signal Specification5/1
  Demux/2 -> Vector Concatenate2/1
  Demux/1 -> Vector Concatenate1/1
  Vector Concatenate2/1 -> Vector Concatenate3/2
  Vector Concatenate1/1 -> Vector Concatenate3/1
  Vector Concatenate3/1 -> F_out/1
  Ground/1 -> Vector Concatenate1/2, Vector Concatenate2/2

== system autolibshared/Vehicle Body 3DOF Single Track/front forces/int ==
  Ground : Ground
  Vector Concatenate1 : Concatenate
  F_out : Outport  VectorParamsAs1DForOutWhenUnconnected=off
  wires:
  Vector Concatenate1/1 -> F_out/1
  Ground/1 -> Vector Concatenate1/1, Vector Concatenate1/2

== system autolibshared/Vehicle Body 3DOF Single Track/front forces/int dual ==
  Ground : Ground
  Vector Concatenate2 : Concatenate  Mode=Multidimensional array  ConcatenateDimension=2
  Vector Concatenate3 : Concatenate  Mode=Multidimensional array  ConcatenateDimension=2
  Vector Concatenate4 : Concatenate  Mode=Multidimensional array
  F_out : Outport  VectorParamsAs1DForOutWhenUnconnected=off
  wires:
  Ground/1 -> Vector Concatenate2/1, Vector Concatenate2/2, Vector Concatenate3/1, Vector Concatenate3/2
  Vector Concatenate4/1 -> F_out/1
  Vector Concatenate3/1 -> Vector Concatenate4/2
  Vector Concatenate2/1 -> Vector Concatenate4/1

== system autolibshared/Vehicle Body 3DOF Single Track/front steer/delta ext ==
  delta_in : Inport  Unit=rad
  Signal Specification1 : SignalSpecification  Unit=rad
  Unit Conversion1 : UnitConversion
  delta_out : Outport  VectorParamsAs1DForOutWhenUnconnected=off
  wires:
  delta_in/1 -> Unit Conversion1/1
  Unit Conversion1/1 -> Signal Specification1/1
  Signal Specification1/1 -> delta_out/1

== system autolibshared/Vehicle Body 3DOF Single Track/front steer/delta ext dual ==
  delta_in : Inport  PortDimensions=2
  Signal Specification1 : SignalSpecification  Unit=rad
  Unit Conversion2 : UnitConversion
  delta_out : Outport  Unit=rad  PortDimensions=2  VectorParamsAs1DForOutWhenUnconnected=off
  wires:
  delta_in/1 -> Unit Conversion2/1
  Unit Conversion2/1 -> Signal Specification1/1
  Signal Specification1/1 -> delta_out/1

== system autolibshared/Vehicle Body 3DOF Single Track/front steer/delta int ==
  Ground : Ground
  delta_out : Outport  VectorParamsAs1DForOutWhenUnconnected=off
  wires:
  Ground/1 -> delta_out/1

== system autolibshared/Vehicle Body 3DOF Single Track/front steer/delta int dual ==
  Constant : Constant  Value=0
  Vector Concatenate4 : Concatenate
  delta_out : Outport  VectorParamsAs1DForOutWhenUnconnected=off
  wires:
  Vector Concatenate4/1 -> delta_out/1
  Constant/1 -> Vector Concatenate4/2, Vector Concatenate4/1

== system autolibshared/Vehicle Body 3DOF Single Track/sigma/no sigma ==
  y : Inport
  Demux : Demux  Outputs=2
  Selector : Selector  InputPortWidth=4  IndexOptions=Index vector (dialog)  Indices=[1,3]  OutputSizes=1
  alpha_f : Outport  VectorParamsAs1DForOutWhenUnconnected=off
  alpha_r : Outport  Port=2  VectorParamsAs1DForOutWhenUnconnected=off
  wires:
  y/1 -> Selector/1
  Selector/1 -> Demux/1
  Demux/1 -> alpha_f/1
  Demux/2 -> alpha_r/1

== system autolibshared/Vehicle Body 3DOF Single Track/sigma/no sigma dual ==
  y : Inport  PortDimensions=8
  Demux : Demux  Outputs=[2,2,4]
  Terminator : Terminator
  alpha_f : Outport  VectorParamsAs1DForOutWhenUnconnected=off
  alpha_r : Outport  Port=2  VectorParamsAs1DForOutWhenUnconnected=off
  wires:
  Demux/3 -> Terminator/1
  Demux/2 -> alpha_r/1
  Demux/1 -> alpha_f/1
  y/1 -> Demux/1

== system autolibshared/Vehicle Body 3DOF Single Track/sigma/sigma ==
  y : Inport
  Constant1 : Constant  Value=sigma_f
  Constant2 : Constant  Value=sigma_r
  Demux : Demux
  relaxation front : Subsystem
  relaxation rear : Subsystem
  alpha_f : Outport  VectorParamsAs1DForOutWhenUnconnected=off
  alpha_r : Outport  Port=2  VectorParamsAs1DForOutWhenUnconnected=off
  wires:
  relaxation front/1(alpha_sig) -> alpha_f/1
  Demux/1 -> relaxation front/1(alpha)
  relaxation rear/1(alpha_sig) -> alpha_r/1
  Demux/4 -> relaxation rear/2(V)
  Demux/2 -> relaxation front/2(V)
  Constant2/1 -> relaxation rear/3(sigma)
  Constant1/1 -> relaxation front/3(sigma)
  y/1 -> Demux/1
  Demux/3 -> relaxation rear/1(alpha)

== system autolibshared/Vehicle Body 3DOF Single Track/sigma/sigma dual ==
  y : Inport  PortDimensions=8
  Constant1 : Constant  Value=sigma_f
  Constant2 : Constant  Value=sigma_r
  Demux : Demux  Outputs=[4,4]
  Demux1 : Demux  Outputs=[2,2]
  Vector Concatenate : Concatenate  NumInputs=4
  relaxation : Subsystem
  alpha_f : Outport  VectorParamsAs1DForOutWhenUnconnected=off
  alpha_r : Outport  Port=2  VectorParamsAs1DForOutWhenUnconnected=off
  wires:
  Demux1/2 -> alpha_r/1
  Demux1/1 -> alpha_f/1
  Vector Concatenate/1 -> relaxation/3(sigma)
  Constant2/1 -> Vector Concatenate/4, Vector Concatenate/3
  Constant1/1 -> Vector Concatenate/1, Vector Concatenate/2
  y/1 -> Demux/1
  Demux/2 -> relaxation/2(V)
  Demux/1 -> relaxation/1(alpha)
  relaxation/1(alpha_sig) -> Demux1/1

== system autolibshared/Vehicle Body 3DOF Single Track/state/xdot ext ==
  xdot : Inport
  xddot_in : Inport  Port=2  PortDimensions=4
  extState : Inport  Port=3
  Integrator : Integrator  InitialConditionSource=external  InitialCondition=[x_o;ydot_o;psi;r_o;x_o;xdot_o]
  Selector : Selector  InputPortWidth=4  IndexOptions=Index vector (dialog)  Indices=[2:4]  OutputSizes=1
  Selector1 : Selector  InputPortWidth=4  IndexOptions=Index vector (dialog)  Indices=[2:4]  OutputSizes=1
  Signal Specification : SignalSpecification  Unit=m/s
  Unit Conversion6 : UnitConversion
  Vector Concatenate : Concatenate
  Vector Concatenate1 : Concatenate
  xddot_out : Outport  VectorParamsAs1DForOutWhenUnconnected=off
  wires:
  Signal Specification/1 -> Vector Concatenate1/1, Vector Concatenate/1
  Unit Conversion6/1 -> Signal Specification/1
  Integrator/1 -> Selector/1
  Vector Concatenate/1 -> Integrator/2
  xdot/1 -> Unit Conversion6/1
  Selector/1 -> Vector Concatenate1/2
  Vector Concatenate1/1 -> xddot_out/1
  xddot_in/1 -> Integrator/1
  extState/1 -> Selector1/1
  Selector1/1 -> Vector Concatenate/2

== system autolibshared/Vehicle Body 3DOF Single Track/state/xdot int ==
  xddot_in : Inport  PortDimensions=4
  extState : Inport  Port=2
  Integrator : Integrator  InitialConditionSource=external  InitialCondition=[x_o;ydot_o;psi;r_o;x_o;xdot_o]
  xddot_out : Outport  VectorParamsAs1DForOutWhenUnconnected=off
  wires:
  Integrator/1 -> xddot_out/1
  xddot_in/1 -> Integrator/1
  extState/1 -> Integrator/2

== system autolibshared/Vehicle Body 3DOF Single Track/wind/wind ext ==
  wind_in : Inport
  Signal Specification1 : SignalSpecification  Unit=m/s
  Unit Conversion5 : UnitConversion
  wind_out : Outport  Unit=m/s  VectorParamsAs1DForOutWhenUnconnected=off
  wires:
  Unit Conversion5/1 -> Signal Specification1/1
  wind_in/1 -> Unit Conversion5/1
  Signal Specification1/1 -> wind_out/1

== system autolibshared/Vehicle Body 3DOF Single Track/wind/wind int ==
  Ground : Ground
  Vector Concatenate1 : Concatenate  NumInputs=3
  wind_out : Outport  Unit=m/s  VectorParamsAs1DForOutWhenUnconnected=off
  wires:
  Vector Concatenate1/1 -> wind_out/1
  Ground/1 -> Vector Concatenate1/3, Vector Concatenate1/2, Vector Concatenate1/1

== system autolibshared/Longitudinal Wheel/Wheel Module/Brakes/Disk Brake ==
  BrkPrs : Inport
  Omega : Inport  Port=2
  Disk Brake : autolibsharedcommon/Disk Brake  disk_abore=disk_abore  num_pads=num_pads  Rm=Rm  mu_kinetic=mu_kinetic
      settings: SourceProductName=Powertrain Blockset  SourceProductBaseCode=PW
  MyBrk : Outport  VectorParamsAs1DForOutWhenUnconnected=off
  wires:
  Disk Brake/1 -> MyBrk/1
  Omega/1 -> Disk Brake/2
  BrkPrs/1 -> Disk Brake/1

== system autolibshared/Longitudinal Wheel/Wheel Module/Brakes/Drum Brake ==
  BrkPrs : Inport
  Omega : Inport  Port=2
  Drum Brake : Subsystem  mask{drum_abore=drum_abore, mu_kinetic=mu_kinetic, drum_a=drum_a, drum_c=drum_c, drum_r=drum_r, drum_theta1=drum_theta1, drum_theta2=drum_theta2}
      mask prompts: drum_abore "Drum brake actuator bore, drum_abore [m]:"; mu_kinetic "Kinetic friction coefficient, mu_kinetic [-]:"; drum_a "Shoe pin to drum center distance, drum_a [m]:"; drum_c "Shoe pin center to force application point distance, drum_c [m]:"; drum_r "Drum internal radius, drum_r [m]:"; drum_theta1 "Shoe pin to pad start angle, drum_theta1 [deg]:"; drum_theta2 "Shoe pin to pad end angle, drum_theta2 [deg]:"
      mask help: Implements a drum brake pressure to torque transformation model based on the drum and shoe geometry parameters provided by the user.
  MyBrk : Outport  VectorParamsAs1DForOutWhenUnconnected=off
  wires:
  BrkPrs/1 -> Drum Brake/1(Brake Pressure)
  Omega/1 -> Drum Brake/2(Wheel angular velocity)
  Drum Brake/1(Brake Torque) -> MyBrk/1

== system autolibshared/Longitudinal Wheel/Wheel Module/Brakes/Mapped Brake ==
  BrkPrs : Inport
  Omega : Inport  Port=2
  Mapped Brake : autolibsharedcommon/Mapped Brake  brake_p_bpt=brake_p_bpt  brake_n_bpt=brake_n_bpt  f_brake_t=f_brake_t
      settings: SourceProductName=Powertrain Blockset  SourceProductBaseCode=PW
  Memory : Memory  InitialCondition=omegao
  MyBrk : Outport  VectorParamsAs1DForOutWhenUnconnected=off
  wires:
  BrkPrs/1 -> Mapped Brake/1
  Mapped Brake/1 -> MyBrk/1
  Omega/1 -> Memory/1
  Memory/1 -> Mapped Brake/2

== system autolibshared/Longitudinal Wheel/Wheel Module/Brakes/No Brake ==
  BrkPrs : Inport
  Omega : Inport  Port=2
  Ground : Ground
  Terminator : Terminator
  Terminator1 : Terminator
  MyBrk : Outport  VectorParamsAs1DForOutWhenUnconnected=off
  wires:
  Omega/1 -> Terminator1/1
  Ground/1 -> MyBrk/1
  BrkPrs/1 -> Terminator/1
